simulink model "Capstone_project_2"  (R2023a)
settings: Solver=VariableStepAuto  StartTime=0.0  StopTime=simtime  MaxStep=0.001  RelTol=1e-3
undefined symbols (not defined in the file): b_1, b_2, F_in, k_1, k_2, m_1, m_2
settings Model: Creator=fycce  LastModifiedBy=fycce
settings DataIOCC: SaveOutput=off  SaveTime=off  ReturnWorkspaceOutputs=off

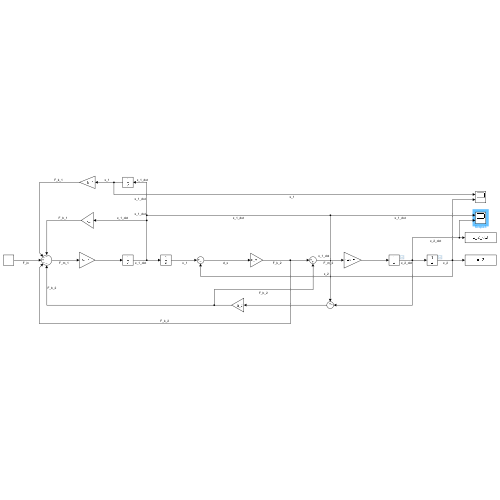
[thumbnail: Simulink's stored preview of the top-level diagram]
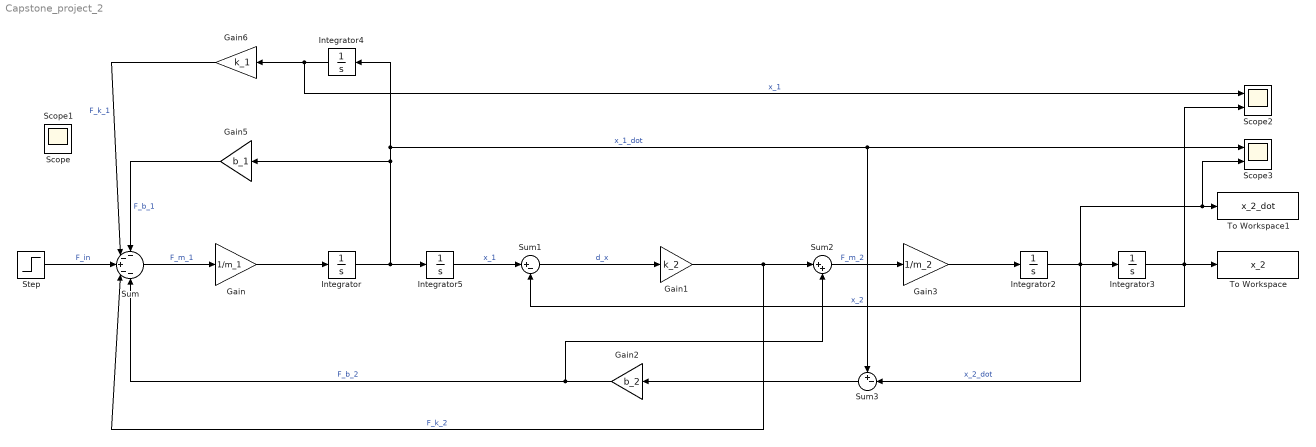
== system Capstone_project_2 ==
  Gain : Gain  Gain=1/m_1
  Gain1 : Gain  Gain=k_2
  Gain2 : Gain  Gain=b_2
  Gain3 : Gain  Gain=1/m_2
  Gain5 : Gain  Gain=b_1
  Gain6 : Gain  Gain=k_1
  Integrator{,2..5} (5 alike) : Integrator
  Scope2 : Scope  NumInputPorts=2
  Scope3 : Scope  NumInputPorts=2
  Step : Step  After=F_in  SampleTime=0
  Sum : Sum  Inputs=--+--
  Sum1 : Sum  Inputs=|+-
  Sum2 : Sum  Inputs=|++
  Sum3 : Sum  Inputs=+-|
  To Workspace : ToWorkspace  VariableName=x_2  SaveFormat=Timeseries  SampleTime=-1
  To Workspace1 : ToWorkspace  VariableName=x_2_dot  SaveFormat=Timeseries  SampleTime=-1
  Scope : Scope
  Scope1 : Scope
  wires:
  Step/1 -> Sum/3  "F_in"
  Sum/1 -> Gain/1  "F_m_1"
  Gain/1 -> Integrator/1
  Integrator/1 -> Integrator5/1, Integrator4/1, Sum3/1, Scope3/1, Gain5/1  "x_1_dot"
  Sum1/1 -> Gain1/1  "d_x"
  Gain1/1 -> Sum2/1, Sum/4  "F_k_2"
  Sum2/1 -> Gain3/1  "F_m_2"
  Gain3/1 -> Integrator2/1
  Integrator2/1 -> Sum3/2, Scope3/2, To Workspace1/1, Integrator3/1  "x_2_dot"
  Integrator3/1 -> Scope2/2, To Workspace/1, Sum1/2  "x_2"
  Gain5/1 -> Sum/1  "F_b_1"
  Integrator4/1 -> Scope2/1, Gain6/1  "x_1"
  Gain6/1 -> Sum/2  "F_k_1"
  Gain2/1 -> Sum2/2, Sum/5  "F_b_2"
  Integrator5/1 -> Sum1/1  "x_1"
  Sum3/1 -> Gain2/1
